simulink model "rasberry"  (R2019b)
settings: Solver=FixedStepAuto  StartTime=0.0  StopTime=10.0  RelTol=1e-3
libraries: embdlinuxlib x1
settings Model: SimulationMode=external  Creator=sbuadu  LastModifiedBy=bhisma
settings SolverCC: PositivePriorityOrder=on
settings DataIOCC: ReturnWorkspaceOutputs=off
settings OptimizationCC: MaxStackSize=64  EfficientTunableParamExpr=on
settings DebuggingCC: ParameterTunabilityLossMsg=error  ArithmeticOperatorsInVariantConditions=warning
settings HardwareCC: ProdBitPerPointer=32  ProdBitPerSizeT=32  ProdBitPerPtrDiffT=32  ProdLargestAtomicInteger=Long  ProdLargestAtomicFloat=Double  ProdWordSize=32  ProdHWDeviceType=ARM Compatible->ARM Cortex
settings SFSimCC: SimUseLocalCustomCode=off  MATLABDynamicMemAlloc=off  CustomCodeUndefinedFunction=UseInterfaceOnly
settings RTWCC: SystemTargetFile=ert.tlc  HardwareBoard=Raspberry Pi  TLCOptions="-aInlineSetEventsForThisBaseRateFcn=TLC_FALSE -aSuppressMultiTaskScheduler=TLC_FALSE  -aRateBasedStepFcn=0"  TemplateMakefile=ert_default_tmf  GenerateReport=on  RTWUseLocalCustomCode=off  Toolchain=GNU GCC Raspberry Pi  IncludeHyperlinkInReport=on  LaunchReport=on  GenerateTraceInfo=on  GenerateTraceReport=on  GenerateTraceReportSl=on  GenerateTraceReportSf=on  GenerateTraceReportEml=on
settings CodeAppCC: ForceParamTrailComments=on  IgnoreCustomStorageClasses=off  OperatorAnnotations=on  SimulinkDataObjDesc=on  SFDataObjDesc=on  MATLABFcnDesc=on  InsertBlockDesc=on  StateflowObjectComments=on  MATLABSourceComments=on
settings ERTTargetCC: MultiwordLength=2048  SupportVariableSizeSignals=on

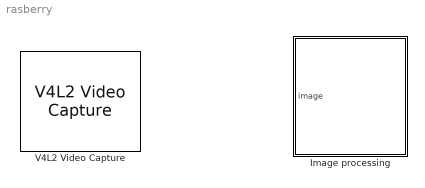
== system rasberry ==
  Image processing : Subsystem
  V4L2 Video Capture : embdlinuxlib/V4L2 Video Capture  m_devName='/dev/video0'  roi=[0, 0, 640, 480]  imSizeSelection=160x120  imSize=[640, 480]  pixelFormat=RGB  pixelOrder=Planar  sampleTime=1/10  simOutput=Colorbars  blockPlatform=Raspberry Pi
      settings: SourceProductName=Simulink Support Package for Raspberry Pi Hardware  SourceProductBaseCode=RASPPI

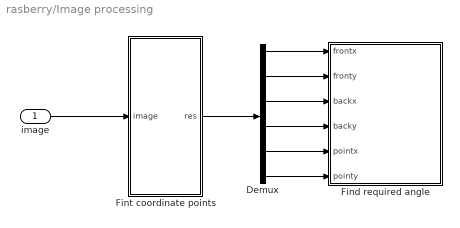
== system rasberry/Image processing ==
  "image " : Inport
  Demux : Demux  Outputs=6
  Find required angle : MATLAB Function  TreatAsAtomicUnit=on
  Fint coordinate points : MATLAB Function  TreatAsAtomicUnit=on
  wires:
  Demux/2 -> Find required angle/2(fronty)
  Demux/4 -> Find required angle/4(backy)
  Demux/1 -> Find required angle/1(frontx)
  Demux/3 -> Find required angle/3(backx)
  Demux/5 -> Find required angle/5(pointx)
  Demux/6 -> Find required angle/6(pointy)
  "image "/1 -> Fint coordinate points/1(image)
  Fint coordinate points/1(res) -> Demux/1

== matlab function rasberry/Image processing/Fint coordinate points ==
  data: image input; res output
function res = findColor( image)

resizeIm = 0.1;

%image = ('double1.jpg');
image = imread(image);
image = imresize(image,resizeIm);
[m,n] = size(image);

red = image(:,:,1);
blue = image(:,:,3);
green = image - red;
greenIntensity = rgb2gray(green);
greenBinary = imbinarize(greenIntensity);
s = regionprops(greenBinary,'centroid');
centroids = cat(1, s.Centroid);
a = regionprops(greenBinary, 'area');
area = cat(1, a.Area);

imshow(greenBinary);
hold on
plot(centroids(:,1),centroids(:,2), 'b*')
hold off


[sortedValues,sortIndex] = sort(area(:),'descend');

if size(area,1) == 2
    frontPos = centroids(sortIndex(1),:)
    backPos = centroids(sortIndex(2),:)
    destination = [0,0];
elseif size(area,1)== 3
    destination = centroids(sortIndex(1),:)
    frontPos = centroids(sortIndex(2),:)
    backPos = centroids(sortIndex(3),:)
else
    error('did not find correct number of green spots');
end
    res = [frontpos, frontpos1, backpos,backpos1, destination,destination1]  ; 

end

== matlab function rasberry/Image processing/Find required angle ==
  data: frontx input; fronty input; backx input; backy input; pointx input; pointy input
function findAngle(frontx, fronty, backx, backy, pointx, pointy)

%%setting the coordinates for the middle of the car 
if frontx < backx
    carx = frontx + abs(backx - frontx)/2; 
else
    carx = backx + abs(backx - frontx)/2; 
end

if fronty < backy
    cary = fronty + abs(backy - fronty)/2; 
else
    cary = backy + abs(backy - fronty)/2;  
end


%%finding the vector between car and destination 
deltax = pointx - carx; 
deltay = pointy-cary; 
delta = [deltax deltay]; 
%%tvector from rotation point to frot of vehicle
betax = frontx - carx;
betay = fronty-cary; 
beta = [betax betay]; 

alpha = atan2(beta(2), beta(1)) - atan2(delta(2), delta(1)); 

alpha = alpha*180/pi; 

if alpha > 180
alpha = alpha - 360; 
end


end
